simulink model "onthebus_fd_alt3"  (R2025b)
settings: Solver=FixedStepAuto  StartTime=0.0  StopTime=inf  RelTol=1e-3  EnableMultiTasking=on
undefined symbols (not defined in the file): position, timestamp, yaw
libraries: px4uORBlib x6, px4Utilslib x3, simulink x2
settings Model: ExtModeTrigDuration=10  Creator=The MathWorks, Inc.  LastModifiedBy=patri
settings SolverCC: AlgebraicLoopSolver=TrustRegion  PositivePriorityOrder=on  MaxZcPerStep=1.0
settings OptimizationCC: UseDivisionForNetSlopeComputation=on  EnhancedBackFolding=on  PassReuseOutputArgsAs=Individual arguments  ZeroExternalMemoryAtStartup=off  ZeroInternalMemoryAtStartup=off  EfficientFloat2IntCast=on  MaxStackSize=64  OptimizeBlockOrder=speed  DifferentSizesBufferReuse=on  OptimizationCustomize=off  EfficientTunableParamExpr=on
settings DebuggingCC: SignalInfNanChecking=warning  ParameterPrecisionLossMsg=none  ParameterTunabilityLossMsg=error  UnconnectedInputMsg=warning  UnconnectedOutputMsg=warning  UnconnectedLineMsg=warning  UniqueDataStoreMsg=error  AssertControl=DisableAll  SubsystemReferenceDiagnosticForUnitTest=warning  ArithmeticOperatorsInVariantConditions=warning
settings HardwareCC: ProdBitPerPointer=32.0  ProdBitPerSizeT=32.0  ProdBitPerPtrDiffT=32.0  ProdLargestAtomicInteger=Long  ProdLargestAtomicFloat=Double  ProdWordSize=32.0  ProdLongLongMode=on  ProdHWDeviceType=ARM Compatible->ARM Cortex
settings ModelReferenceCC: EnableRefExpFcnMdlSchedulingChecks=on
settings SFSimCC: CompileTimeRecursionLimit=0.0  EnableRuntimeRecursion=off  MATLABDynamicMemAlloc=off  SimTargetLang=C++  SimDLTargetLibrary=mkl-dnn
settings RTWCC: SystemTargetFile=ert.tlc  HardwareBoard=PX4 Host Target  TLCOptions="-aInlineSetEventsForThisBaseRateFcn=TLC_FALSE -aSuppressMultiTaskScheduler=TLC_FALSE  -aRateBasedStepFcn=0"  TemplateMakefile=ert_default_tmf  GenerateReport=on  Toolchain=GNU Tools for PX4 Autopilots  IncludeHyperlinkInReport=on  LaunchReport=on  PortableWordSizes=on  TargetLang=C++  GenerateTraceInfo=on  GenerateTraceReport=on  GenerateTraceReportSl=on  GenerateTraceReportSf=on  GenerateTraceReportEml=on  GPUComputeCapability=3.5  DLArmComputeVersion=19.05  Description=Embedded Coder
settings CodeAppCC: ForceParamTrailComments=on  IgnoreCustomStorageClasses=off  IgnoreTestpoints=on  OperatorAnnotations=on  SimulinkDataObjDesc=on  SFDataObjDesc=on  MATLABFcnDesc=on  InsertBlockDesc=on
settings ERTTargetCC: ExtModeTransport=2.0  ExtModeStaticAlloc=on  ExtModeMexFile=ext_xcp  ExtModeIntrfLevel=Level2 - Open  InlinedParameterPlacement=Hierarchical  SuppressUnreachableDefaultCases=off  EnableSignedLeftShifts=off  EnableSignedRightShifts=off  UtilityFuncGeneration=Shared location  SupportNonFinite=off  ParenthesesLevel=Standards  CastingMode=Standards

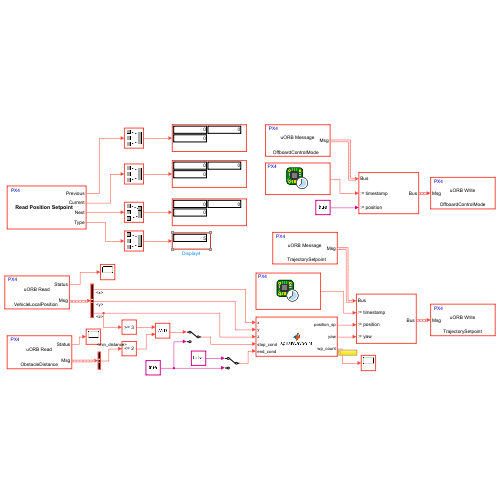
[thumbnail: Simulink's stored preview of the top-level diagram]
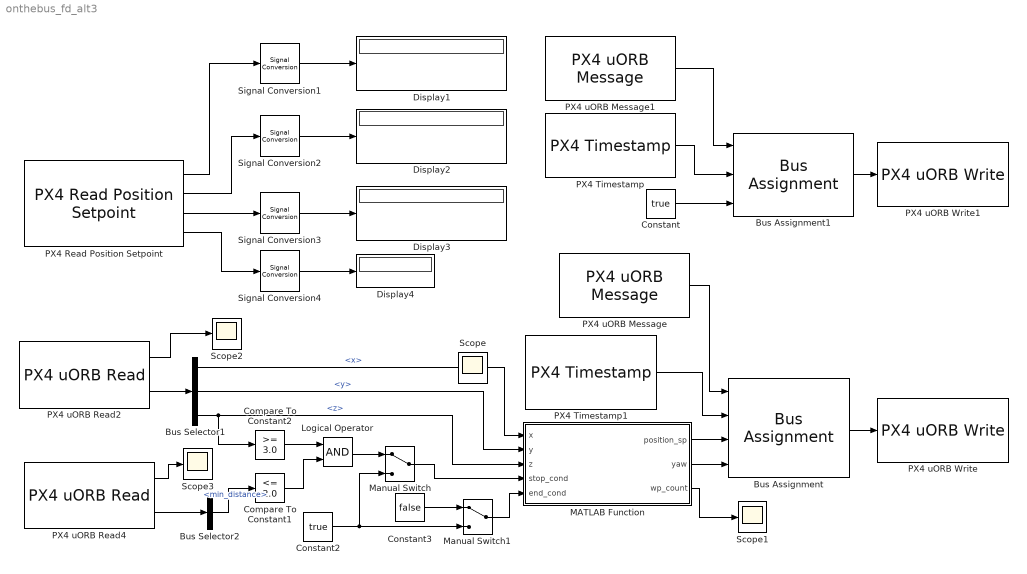
== system onthebus_fd_alt3 ==
  Bus Assignment : BusAssignment  AssignedSignals=timestamp,position,yaw
  Bus Assignment1 : BusAssignment  AssignedSignals=timestamp,position
  Bus Selector1 : BusSelector  OutputSignals=x,y,z
  Bus Selector2 : BusSelector  OutputSignals=min_distance
  Compare To Constant1 : simulink/Logic and Bit Operations/Compare To Constant  relop=<=  const=2.0  OutDataTypeStr=boolean
  Compare To Constant2 : simulink/Logic and Bit Operations/Compare To Constant  relop=>=  const=3.0  OutDataTypeStr=boolean
  Constant : Constant  Value=true
  Constant2 : Constant  Value=true
  Constant3 : Constant  Value=false
  Display{1..4} (4 alike) : Display
  Logical Operator : Logic  AllPortsSameDT=off  OutDataTypeStr=boolean
  MATLAB Function : MATLAB Function  TreatAsAtomicUnit=on
  Manual Switch : ManualSwitch
  Manual Switch1 : ManualSwitch
  PX4 Read Position Setpoint : px4Utilslib/PX4 Read Position Setpoint  coordinateFrame=Local Coordinates (NED)  SampleTime=.05  positionSetpointBus=off  trajectoryWaypointsBus=off  onboardFailsafeFlag=off  onboardEnableStatus=off
  PX4 Timestamp : px4Utilslib/PX4 Timestamp  SampleTime=.05
  PX4 Timestamp1 : px4Utilslib/PX4 Timestamp  SampleTime=.05
  PX4 uORB Message : px4uORBlib/PX4 uORB Message  uORBTopic=TrajectorySetpoint  SampleTime=.05  selectInstance=TrajectorySetpoint
  PX4 uORB Message1 : px4uORBlib/PX4 uORB Message  uORBTopic=OffboardControlMode  SampleTime=.05  selectInstance=OffboardControlMode
  PX4 uORB Read2 : px4uORBlib/PX4 uORB Read  uORBTopic=VehicleLocalPosition  selectInstance=vehicle_local_position  SampleTime=.05  BlockingMode=off  BlockTimeout=1e-3
  PX4 uORB Read4 : px4uORBlib/PX4 uORB Read  uORBTopic=ObstacleDistance  selectInstance=obstacle_distance  SampleTime=.05  BlockingMode=off  BlockTimeout=1e-3
  PX4 uORB Write : px4uORBlib/PX4 uORB Write  uORBTopic=TrajectorySetpoint  selectInstance=TrajectorySetpoint  MessageQueueLen=1
  PX4 uORB Write1 : px4uORBlib/PX4 uORB Write  uORBTopic=OffboardControlMode  selectInstance=OffboardControlMode  MessageQueueLen=1
  Scope{,1..3} (4 alike) : Scope
      Scope1 settings: DataLoggingVariableName=ScopeData2
      Scope3 settings: DataLoggingVariableName=ScopeData3
      Scope settings: ActiveDisplayYMinimum=-1  ActiveDisplayYMaximum=1
  Signal Conversion{1..4} (4 alike) : SignalConversion  OverrideOpt=off
  wires:
  PX4 Read Position Setpoint/2 -> Signal Conversion2/1
  Constant/1 -> Bus Assignment1/3
  PX4 Read Position Setpoint/3 -> Signal Conversion3/1
  PX4 Read Position Setpoint/4 -> Signal Conversion4/1
  Signal Conversion4/1 -> Display4/1
  Signal Conversion3/1 -> Display3/1
  Signal Conversion2/1 -> Display2/1
  Signal Conversion1/1 -> Display1/1
  PX4 Read Position Setpoint/1 -> Signal Conversion1/1
  PX4 Timestamp/1 -> Bus Assignment1/2
  Bus Assignment1/1 -> PX4 uORB Write1/1
  PX4 uORB Message/1 -> Bus Assignment/1
  PX4 Timestamp1/1 -> Bus Assignment/2
  MATLAB Function/1(position_sp) -> Bus Assignment/3
  MATLAB Function/2(yaw) -> Bus Assignment/4
  MATLAB Function/3(wp_count) -> Scope1/1
  Bus Assignment/1 -> PX4 uORB Write/1
  PX4 uORB Message1/1 -> Bus Assignment1/1
  PX4 uORB Read2/2 -> Bus Selector1/1
  Bus Selector1/1 -> MATLAB Function/1(x)  "<x>"
  Bus Selector1/2 -> MATLAB Function/2(y)  "<y>"
  Bus Selector1/3 -> MATLAB Function/3(z), Compare To Constant2/1  "<z>"
  PX4 uORB Read4/2 -> Bus Selector2/1
  Bus Selector2/1 -> Compare To Constant1/1  "<min_distance>"
  PX4 uORB Read2/1 -> Scope2/1
  PX4 uORB Read4/1 -> Scope3/1
  Manual Switch/1 -> MATLAB Function/4(stop_cond)
  Manual Switch1/1 -> MATLAB Function/5(end_cond)
  Constant2/1 -> Manual Switch/2, Manual Switch1/2
  Logical Operator/1 -> Manual Switch/1
  Compare To Constant2/1 -> Logical Operator/1
  Compare To Constant1/1 -> Logical Operator/2
  Constant3/1 -> Manual Switch1/1

== matlab function onthebus_fd_alt3/MATLAB Function ==
  data: position_sp output; x input; yaw output; y input; z input; stop_cond input; wp_count output; end_cond input
function [position_sp, yaw, wp_count] = spiralWaypoint(x, y, z, stop_cond, end_cond)

%% Persistent state
persistent waypoints idx initialized wp_count_p home_x home_y mission_done hold_pos holding

MAX_WP = 50;     
base = 2.0;      
alt = -4.0;      

%% Init
if isempty(initialized)

    hold_pos = [0 0 alt];

    waypoints = zeros(MAX_WP, 3);

    % Save home position
    home_x = x;
    home_y = y;

    % Generate square spiral
    px = 0; 
    py = 0;
    step = base;

    waypoints(1,:) = [home_x, home_y, alt];

    for k = 1:(MAX_WP-1)
        switch mod(k-1,4)
            case 0, px = px + step;
            case 1, py = py + step;
            case 2, px = px - step;
            case 3, py = py - step;
        end

        waypoints(k+1,:) = [home_x + py, home_y + px, alt];

        if mod(k,2) == 0
            step = step + base;
        end
    end

    idx = 1;
    wp_count_p = 0;
    mission_done = false;
    holding = false;
    initialized = true;
end

pos_ned = [x y z];

%% ================= STOP (HIGHEST PRIORITY) =================
if stop_cond && ~holding
    hold_pos = double(pos_ned);   % capture current position
    holding = true;
end

if stop_cond && end_cond
    mission_done = true;
end

if holding && ~mission_done
    position_sp = single(hold_pos);

    dir = hold_pos - pos_ned;
    if norm(dir) > 0.01
        yaw = atan2(dir(2), dir(1));
    else
        yaw = single(0);
    end

    wp_count = wp_count_p;
    return;
end

if mission_done
    target = [home_x, home_y, alt];

    position_sp = single(target);

    dir = target - pos_ned;
    if norm(dir) > 0.01
        yaw = atan2(dir(2), dir(1));
    else
        yaw = single(0);
    end

    wp_count = wp_count_p;
    return;
end
%% ===========================================================

%% Normal waypoint tracking
target = waypoints(idx,:);

tolerance = 0.3;

if norm(pos_ned - target) < tolerance
    wp_count_p = wp_count_p + 1;
    if idx < MAX_WP
        idx = idx + 1;
    end
end

target = waypoints(idx,:);

position_sp = single(target);

dir = target - pos_ned;
yaw = atan2(dir(2), dir(1));

wp_count = wp_count_p;

end
